simulink model "cart_pole_sim_LQR_v2"  (R2026a)
settings: Solver=ode23tb  StartTime=0.01  StopTime=60  MaxStep=0.005  MinStep=1e-6  AbsTol=1e-5
settings Model: Creator=heber  LastModifiedBy=heber

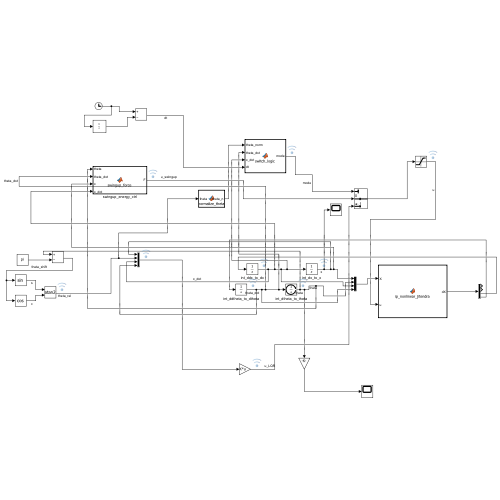
[thumbnail: Simulink's stored preview of the top-level diagram]
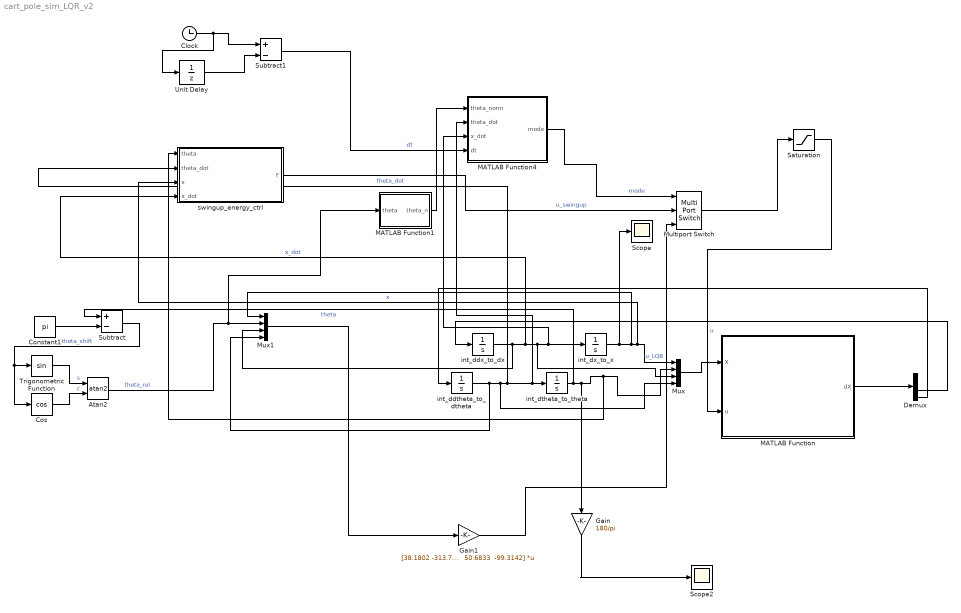
== system cart_pole_sim_LQR_v2 ==
  Atan2 : Trigonometry  Operator=atan2
  Clock : Clock
  Constant1 : Constant  Value=pi
  Cos : Trigonometry  Operator=cos
  Demux : Demux
  Gain : Gain  Gain=180/pi
  Gain1 : Gain  Gain="[38.1802 -313.7776   50.6833  -99.3142]"  Multiplication=Matrix(K*u)
  MATLAB Function : MATLAB Function  TreatAsAtomicUnit=on
  MATLAB Function1 : MATLAB Function  TreatAsAtomicUnit=on
  MATLAB Function4 : MATLAB Function  TreatAsAtomicUnit=on  SystemSampleTime=0.01
  Multiport Switch : MultiPortSwitch  DataPortOrder=Zero-based contiguous  Inputs=2  zeroidx=on  SaturateOnIntegerOverflow=off  InputSameDT=off
  Mux : Mux
  Mux1 : Mux
  Saturation : Saturate  UpperLimit=30  LowerLimit=-30
  Scope : Scope
      settings: ActiveDisplayYMinimum=-0.21164734329640614  ActiveDisplayYMaximum=0.2596236519735593
  Scope2 : Scope
      settings: ActiveDisplayYMinimum=-540.65535935400294  ActiveDisplayYMaximum=495.82439944134182  DataLoggingVariableName=ScopeData2
  Subtract : Sum  Inputs=+-
  Subtract1 : Sum  Inputs=+-
  Trigonometric Function : Trigonometry
  Unit Delay : UnitDelay  SampleTime=-1
  int_ddtheta_to_dtheta : Integrator  ContinuousStateAttributes='dtheta'
  int_ddx_to_dx : Integrator  ContinuousStateAttributes='dx'
  int_dtheta_to_theta : Integrator  InitialCondition=0.05  WrapState=on  ContinuousStateAttributes='theta'
  int_dx_to_x : Integrator  ContinuousStateAttributes='x'
  swingup_energy_ctrl : MATLAB Function  TreatAsAtomicUnit=on
  wires:
  int_ddx_to_dx/1 -> swingup_energy_ctrl/4(x_dot), MATLAB Function4/3(x_dot), int_dx_to_x/1, Mux/3, Mux1/3  "x_dot"
  int_ddtheta_to_dtheta/1 -> swingup_energy_ctrl/2(theta_dot), MATLAB Function4/2(theta_dot), int_dtheta_to_theta/1, Mux/4, Mux1/4  "theta_dot"
  int_dx_to_x/1 -> Mux1/1, swingup_energy_ctrl/3(x), Mux/1, Scope/1  "x"
  int_dtheta_to_theta/1 -> Subtract/1, Gain/1, swingup_energy_ctrl/1(theta), Mux/2  "theta"
  Mux/1 -> MATLAB Function/1(X)
  MATLAB Function/1(dX) -> Demux/1
  Demux/4 -> int_ddtheta_to_dtheta/1
  Demux/3 -> int_ddx_to_dx/1
  Gain/1 -> Scope2/1
  Mux1/1 -> Gain1/1
  Gain1/1 -> Multiport Switch/3  "u_LQR"
  swingup_energy_ctrl/1(F) -> Multiport Switch/2  "u_swingup"
  Saturation/1 -> MATLAB Function/2(u)  "u"
  MATLAB Function1/1(theta_n) -> MATLAB Function4/1(theta_norm)
  Subtract/1 -> Cos/1, Trigonometric Function/1  "theta_shift"
  Constant1/1 -> Subtract/2
  Trigonometric Function/1 -> Atan2/1  "s"
  Cos/1 -> Atan2/2  "c"
  Atan2/1 -> MATLAB Function1/1(theta), Mux1/2  "theta_rel"
  MATLAB Function4/1(mode) -> Multiport Switch/1  "mode"
  Multiport Switch/1 -> Saturation/1
  Clock/1 -> Unit Delay/1, Subtract1/1
  Unit Delay/1 -> Subtract1/2
  Subtract1/1 -> MATLAB Function4/4(dt)  "dt"

== matlab function cart_pole_sim_LQR_v2/MATLAB Function ==
  data: X input; dX output; u input
function dX = ip_nonlinear(X,u)

    % State order (must match Simulink):
    % X(1) = x
    % X(2) = theta
    % X(3) = x_dot
    % X(4) = theta_dot

    dX = zeros(4,1);   % REQUIRED FOR SIMULINK DIMENSION RESOLUTION

    x      = X(1);
    theta  = X(2);
    dx     = X(3);
    dtheta = X(4);

    % ---------------------------------------------------------
    % Updated Physical Parameters (point-mass model)
    % ---------------------------------------------------------
    m  = 0.2;        % pendulum mass [kg]
    M  = 0.8;        % cart mass [kg]
    L  = 0.75;        % pendulum length [m] (pivot to mass)

    % Inertia for point mass at distance L
    I  = m * L^2;    % [kg*m^2]

    % Friction
    B  = 0.01;       % pivot damping [N*m*s]
    C  = 2.0;        % cart viscous friction [N*s/m]

    % Gravity
    g  = 9.81;

    % ---------------------------------------------------------
    % Dynamics
    % ---------------------------------------------------------
    s = sin(theta);
    c = cos(theta);

    % Mass matrix
    A11 = M + m;
    A12 = m * L * c;
    A21 = A12;
    A22 = I + m * L^2;

    % RHS
    b1 = u - C*dx - m * L * dtheta^2 * s;
    b2 = -B*dtheta - m * g * L * s;

    % Solve for accelerations
    den = A11*A22 - A12*A21;
    ddx     = ( A22*b1 - A12*b2 ) / den;
    ddtheta = (-A21*b1 + A11*b2 ) / den;

    % Output derivative vector (must match Simulink integrators):
    dX(1) = dx;
    dX(2) = dtheta;
    dX(3) = ddx;
    dX(4) = ddtheta;

end

== matlab function cart_pole_sim_LQR_v2/swingup_energy_ctrl ==
  data: theta input; F output; theta_dot input; x input; x_dot input
function F = swingup_force(theta, theta_dot, x, x_dot)
%#codegen
m = 0.2;
M = 0.6;
L = 0.75;
g = 9.81;

I  = m * L^2;
Bv = 0.01;
C  = 2.0;

% ===================== TUNING =====================
k_swing = 2;
n       = 0.95;
Fmax    = 30;

% mild cart centering
kx  = 0.6;
kdx = 0.2;

% ===================== ENERGY =========================
E_pot = m*g*L*(1 - cos(theta));
E_kin = 0.5*(I + m*L^2)*theta_dot^2;
E     = E_pot + E_kin;

E_r   = 2*m*g*L;

% Smooth sign
s = (theta_dot * cos(theta));

% Desired acceleration from energy error
accel_raw = 2*(E - E_r) * s;

% Smooth saturation of accel
accel = max(-n*g, min(n*g, accel_raw));
accel = k_swing * accel;

% ===================== ANGLE-DEPENDENT SHAPING (NEW) =====================
% Gradual reduction of accel as pole approaches horizontal
p      = 0;      % smoothness / steepness (try 2, then 3 or 4)
alpha  = 0.0;    % minimum scaling near horizon (0 = kill accel, 1 = no reduction)

c      = cos(theta);
w_theta = alpha + (1 - alpha) * (c^2)^p;
accel   = w_theta * accel;


% ===================== FEEDBACK LINEARIZATION =========
den = (I + m*L^2);

u_swing = (M+m)*accel ...
          - m*L*(theta_dot^2)*sin(theta) ...
          - m*L*cos(theta) * ( (Bv*theta_dot + m*L*accel*cos(theta) + m*g*L*sin(theta)) / den ) ...
          - C*x_dot;

% ===================== MILD CART CENTERING =============
uC = -kx * x - kdx * x_dot;

% ===================== TOTAL FORCE =====================
F = u_swing + uC;
F = max(min(F, Fmax), -Fmax);

end

== matlab function cart_pole_sim_LQR_v2/MATLAB Function1 ==
  data: theta input; theta_n output
function theta_n = normalize_theta(theta)
    theta_n = mod(theta, 2*pi);
end

== matlab function cart_pole_sim_LQR_v2/MATLAB Function4 ==
  data: theta_norm input; mode output; theta_dot input; x_dot input; dt input
function mode = switch_logic(theta_norm, theta_dot, x_dot, dt)

persistent prev_mode t_ready
if isempty(prev_mode), prev_mode = 0; end
if isempty(t_ready),  t_ready  = 0; end

th = abs(theta_norm);
w  = theta_dot;

% ============================================================
% LQR activation thresholds
% ============================================================
ENTER_LQR = 0.12;     % ~7 deg
W_THRESH  = 1;      % angular velocity threshold (rad/s)
DWELL     = 0.03;    % dwell time (s)

% ============================================================
% NO EXIT CONDITION — LQR IS ABSORBING
% ============================================================
if prev_mode == 1
    mode = 1;
    return
end

% ============================================================
% ENTRY CONDITIONS (Swing-up → LQR)
% ============================================================
ang_ok = (th < ENTER_LQR);
w_ok   = (abs(w) < W_THRESH);

if ang_ok && w_ok
    t_ready = t_ready + dt;
    if t_ready >= DWELL
        prev_mode = 1;
    end
else
    t_ready = 0;
end

mode = prev_mode;
end
